simulink model "Unknown_Terrain_BOTS"  (R2018b)
settings: Solver=VariableStepAuto  StartTime=0.0  StopTime=10.0  RelTol=1e-3
model workspace: external: MATLAB File F:\Projects\Relative Localiztion\CAD models\Simulation\Unknown_Terrain_BOTS_DataFile.m (data not in the file)
values from neighbouring files (symbols this model uses):
  BOT1_pos = zeros(3,length(t))    [Tetrahedron_Based_Relative_Localization.m]
  bot1_transmitted = zeros(3,length(t))    [Transmission_Channal.m]
  BOT2_pos = zeros(3,length(t))    [Tetrahedron_Based_Relative_Localization.m]
  bot2_transmitted = zeros(3,length(t))    [Transmission_Channal.m]
  BOT3_pos = zeros(3,length(t))    [Tetrahedron_Based_Relative_Localization.m]
  bot3_transmitted = zeros(3,length(t))    [Transmission_Channal.m]
  BOT4_pos = zeros(3,length(t))    [Tetrahedron_Based_Relative_Localization.m]
  bot4_transmitted = zeros(3,length(t))    [Transmission_Channal.m]
undefined symbols (not defined in the file or in its folder): smiData, X, Y, Z
libraries: simulink x60, sm_lib x29, nesl_utility x25
(part 1 of 2)
settings Model: Creator=Yogesh  LastModifiedBy=Yogesh

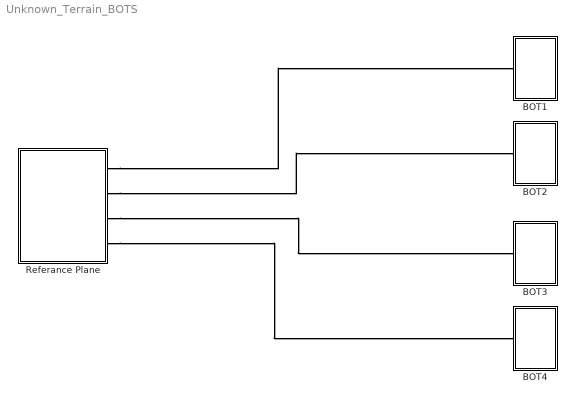
== system Unknown_Terrain_BOTS ==
  BOT1 : Subsystem
  BOT2 : Subsystem
  BOT3 : Subsystem
  BOT4 : Subsystem
  Referance Plane : Subsystem
  connections:
  Referance Plane/RConn1 -- BOT1/LConn1
  Referance Plane/RConn2 -- BOT2/LConn1
  Referance Plane/RConn3 -- BOT3/LConn1
  Referance Plane/RConn4 -- BOT4/LConn1

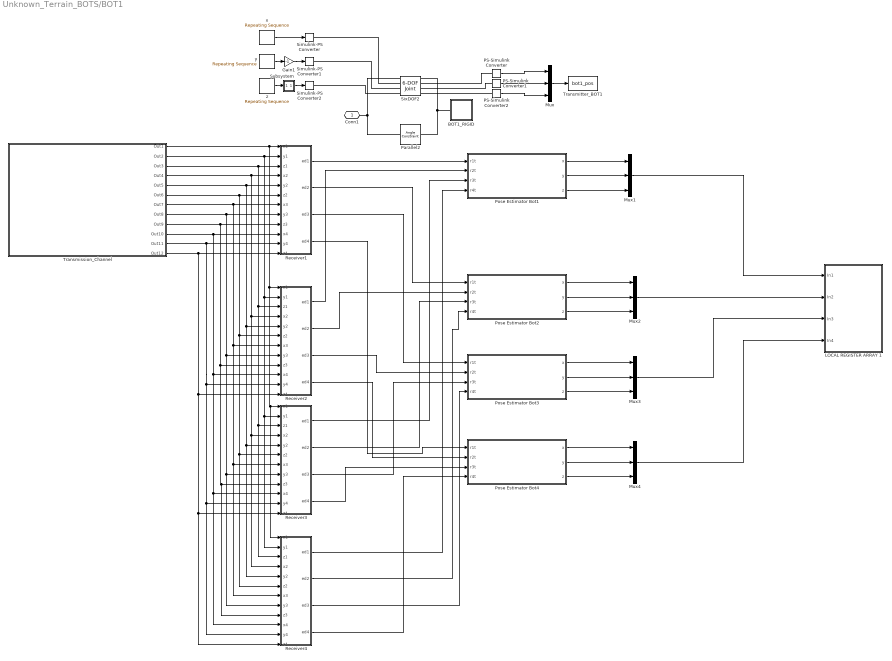
== system Unknown_Terrain_BOTS/BOT1 ==
  BOT1_RIGID : Subsystem
  Gain1 : Gain  Gain=-1
  LOCAL REGISTER ARRAY 1 : Subsystem
  Mux{,1..4} (5 alike) : Mux  Inputs=3
  PS-Simulink Converter : nesl_utility/PS-Simulink Converter  PhysicalDomain=network_engine_domain  SubClassName=ps_output  LeftPortType=input  RightPortType=output  PseudoPeriodic=off  Frequencies=[]  Unit=m  AffineConversion=off
  PS-Simulink Converter1 : nesl_utility/PS-Simulink Converter  PhysicalDomain=network_engine_domain  SubClassName=ps_output  LeftPortType=input  RightPortType=output  PseudoPeriodic=off  Frequencies=[]  Unit=m  AffineConversion=off
  PS-Simulink Converter2 : nesl_utility/PS-Simulink Converter  PhysicalDomain=network_engine_domain  SubClassName=ps_output  LeftPortType=input  RightPortType=output  PseudoPeriodic=off  Frequencies=[]  Unit=m  AffineConversion=off
  Parallel2 : sm_lib/Constraints/Angle Constraint  ConstraintType=Parallel  Angle=45  AngleUnits=deg  SenseSignedTorqueMagnitude=off  SenseTorque=off  SenseForce=off  WrenchDir=FollowerOnBase  WrenchFrame=BaseFrame
      settings: SourceProductName=Simscape Multibody  SourceProductBaseCode=MS
  Pose Estimator Bot1 : MATLAB Function  TreatAsAtomicUnit=on
  Pose Estimator Bot2 : MATLAB Function  TreatAsAtomicUnit=on
  Pose Estimator Bot3 : MATLAB Function  TreatAsAtomicUnit=on
  Pose Estimator Bot4 : MATLAB Function  TreatAsAtomicUnit=on
  Receiver1 : MATLAB Function  TreatAsAtomicUnit=on
  Receiver2 : MATLAB Function  TreatAsAtomicUnit=on
  Receiver3 : MATLAB Function  TreatAsAtomicUnit=on
  Receiver4 : MATLAB Function  TreatAsAtomicUnit=on
  Simulink-PS Converter : nesl_utility/Simulink-PS Converter  PhysicalDomain=network_engine_domain  SubClassName=ps_input  LeftPortType=input  RightPortType=output  PseudoPeriodic=off  Frequencies=[]  NoiseDistribution=none  NoiseParameters=[]  Unit=m  AffineConversion=off  FilteringAndDerivatives=filter  SimscapeFilterOrder=2  InputFilterTimeConstant=0.001  UdotUserProvided=0
  Simulink-PS Converter1 : nesl_utility/Simulink-PS Converter  PhysicalDomain=network_engine_domain  SubClassName=ps_input  LeftPortType=input  RightPortType=output  PseudoPeriodic=off  Frequencies=[]  NoiseDistribution=none  NoiseParameters=[]  Unit=m  AffineConversion=off  FilteringAndDerivatives=filter  SimscapeFilterOrder=2  InputFilterTimeConstant=0.001  UdotUserProvided=0
  Simulink-PS Converter2 : nesl_utility/Simulink-PS Converter  PhysicalDomain=network_engine_domain  SubClassName=ps_input  LeftPortType=input  RightPortType=output  PseudoPeriodic=off  Frequencies=[]  NoiseDistribution=none  NoiseParameters=[]  Unit=m  AffineConversion=off  FilteringAndDerivatives=filter  SimscapeFilterOrder=2  InputFilterTimeConstant=0.001  UdotUserProvided=0
  SixDOF2 : sm_lib/Joints/6-DOF Joint  SenseConstraintForce=off  SenseConstraintForceX=off  SenseConstraintForceY=off  SenseConstraintForceZ=off  SenseConstraintTorque=off  SenseConstraintTorqueX=off  SenseConstraintTorqueY=off  SenseConstraintTorqueZ=off  SenseTotalForce=off  SenseTotalForceX=off  SenseTotalForceY=off  SenseTotalForceZ=off  SenseTotalTorque=off  SenseTotalTorqueX=off  SenseTotalTorqueY=off  SenseTotalTorqueZ=off  CompositeWrenchDir=FollowerOnBase  CompositeWrenchFrame=BaseFrame  PxEquilibriumPosition=0  PxEquilibriumPositionUnits=m  PxSpringStiffness=0  PxSpringStiffnessUnits=N/m  PxDampingCoefficient=0  PxDampingCoefficientUnits=N/(m/s)  PxTorqueActuationMode=ComputedTorque  PxMotionActuationMode=InputMotion  PxSensePosition=on  PxSenseVelocity=off  PxSenseAcceleration=off  PxSenseTorqueForce=off  PxPositionTargetSpecify=on  PxPositionTargetPriority=Low  PxPositionTargetValue=smiData.SixDofJoint(3).Px.Pos  PxPositionTargetValueUnits=in  PxVelocityTargetSpecify=off  PxVelocityTargetPriority=High  PxVelocityTargetValue=0  PxVelocityTargetValueUnits=m/s  PyEquilibriumPosition=0  PyEquilibriumPositionUnits=m  PySpringStiffness=0  PySpringStiffnessUnits=N/m  PyDampingCoefficient=0  PyDampingCoefficientUnits=N/(m/s)  PyTorqueActuationMode=ComputedTorque  PyMotionActuationMode=InputMotion  PySensePosition=on  PySenseVelocity=off  PySenseAcceleration=off  PySenseTorqueForce=off  PyPositionTargetSpecify=on  PyPositionTargetPriority=Low  PyPositionTargetValue=smiData.SixDofJoint(3).Py.Pos  PyPositionTargetValueUnits=in  PyVelocityTargetSpecify=off  PyVelocityTargetPriority=High  PyVelocityTargetValue=0  PyVelocityTargetValueUnits=m/s  PzEquilibriumPosition=0  PzEquilibriumPositionUnits=m  PzSpringStiffness=0  PzSpringStiffnessUnits=N/m  PzDampingCoefficient=0  PzDampingCoefficientUnits=N/(m/s)  PzTorqueActuationMode=ComputedTorque  PzMotionActuationMode=InputMotion  PzSensePosition=on  PzSenseVelocity=off  PzSenseAcceleration=off  PzSenseTorqueForce=off  PzPositionTargetSpecify=on  PzPositionTargetPriority=Low  PzPositionTargetValue=smiData.SixDofJoint(3).Pz.Pos  PzPositionTargetValueUnits=in  PzVelocityTargetSpecify=off  PzVelocityTargetPriority=High  PzVelocityTargetValue=0  PzVelocityTargetValueUnits=m/s  SphDefPosRotationMethod=None  SphDefPosRotationAngleUnits=deg  SphDefPosRotationStandardAxis=+Z  SphDefPosRotationAngle=0.0  SphDefPosRotationArbitraryAxis=[0 0 1]  SphDefPosFollAlignAxisA=+X  SphDefPosBaseAlignAxisA=+Y  SphDefPosFollAlignAxisB=+Y  SphDefPosBaseAlignAxisB=+Z  SphDefPosRotationSequenceAxes=FollowerAxes  SphDefPosRotationSequence=XYX  SphDefPosRotationSequenceAngles=[0 0 0]  SphDefPosRotationSequenceAnglesUnits=deg  SphDefPosRotationMatrix=[1 0 0; 0 1 0; 0 0 1]  SphEqPosRotationMethod=None  SphEqPosRotationAngleUnits=deg  SphEqPosRotationStandardAxis=+Z  SphEqPosRotationAngle=0.0  SphEqPosRotationArbitraryAxis=[0 0 1]  SphEqPosFollAlignAxisA=+X  SphEqPosBaseAlignAxisA=+Y  SphEqPosFollAlignAxisB=+Y  SphEqPosBaseAlignAxisB=+Z  SphEqPosRotationSequenceAxes=FollowerAxes  SphEqPosRotationSequence=XYX  SphEqPosRotationSequenceAngles=[0 0 0]  SphEqPosRotationSequenceAnglesUnits=deg  SphEqPosRotationMatrix=[1 0 0; 0 1 0; 0 0 1]  SphSpringStiffness=0  SphSpringStiffnessUnits=N*m/rad  SphDampingCoefficient=0  SphDampingCoefficientUnits=N*m/(rad/s)  SphActuateTorqueX=off  SphActuateTorqueY=off  SphActuateTorqueZ=off  SphActuateTorque=off  SphTorqueActuationMode=NoTorque  SphMotionActuationMode=ComputedMotion  SphActuationFrame=BaseFrame  SphSensePosition=off  SphSenseVelocityX=off  SphSenseVelocityY=off  SphSenseVelocityZ=off  SphSenseVelocity=off  SphSenseAccelerationX=off  SphSenseAccelerationY=off  SphSenseAccelerationZ=off  SphSenseAcceleration=off  SphSenseTorqueX=off  SphSenseTorqueY=off  SphSenseTorqueZ=off  SphSenseTorqueForce=off  SphSensingFrame=FollowerFrame  SphPositionTargetRotationMethod=ArbitraryAxis  SphPositionTargetRotationAngleUnits=deg  SphPositionTargetRotationStandardAxis=+Z  SphPositionTargetRotationAngle=smiData.SixDofJoint(3).S.Pos.Angle  SphPositionTargetRotationArbitraryAxis=smiData.SixDofJoint(3).S.Pos.Axis  SphPositionTargetFollAlignAxisA=+X  SphPositionTargetBaseAlignAxisA=+Y  SphPositionTargetFollAlignAxisB=+Y  SphPositionTargetBaseAlignAxisB=+Z  SphPositionTargetRotationSequenceAxes=FollowerAxes  SphPositionTargetRotationSequence=XYX  SphPositionTargetRotationSequenceAngles=[0 0 0]  SphPositionTargetRotationSequenceAnglesUnits=deg  SphPositionTargetRotationMatrix=[1 0 0; 0 1 0; 0 0 1]  SphPositionTargetSpecify=on  SphPositionTargetPriority=Low  SphVelocityTargetValue=[0 0 0]  SphVelocityTargetValueUnits=deg/s  SphVelocityTargetSpecify=off  SphVelocityTargetPriority=High  SphVelocityTargetInFollowerFrame=on
  Subsystem : Subsystem
  Transmission_Channel : Subsystem
  Transmitter_BOT1 : ToWorkspace  VariableName=bot1_pos  SampleTime=-1
  x : simulink/Sources/Repeating Sequence  rep_seq_t=t  rep_seq_y=BOT1_pos(1,:)
  y : simulink/Sources/Repeating Sequence  rep_seq_t=t  rep_seq_y=BOT1_pos(2,:)
  z : simulink/Sources/Repeating Sequence  rep_seq_t=t  rep_seq_y=BOT1_pos(3,:)
  Conn1 : PMIOPort  Side=Left
  wires:
  y/1 -> Gain1/1
  z/1 -> Subsystem/1(1)
  Subsystem/1(2) -> Simulink-PS Converter2/1
  x/1 -> Simulink-PS Converter/1
  Gain1/1 -> Simulink-PS Converter1/1
  Mux/1 -> Transmitter_BOT1/1
  PS-Simulink Converter/1 -> Mux/1
  PS-Simulink Converter1/1 -> Mux/2
  PS-Simulink Converter2/1 -> Mux/3
  Receiver4/4(ed4) -> Pose Estimator Bot4/4(r4t)
  Pose Estimator Bot4/1(x) -> Mux4/1
  Pose Estimator Bot3/3(z) -> Mux3/3
  Pose Estimator Bot1/2(y) -> Mux1/2
  Pose Estimator Bot2/2(y) -> Mux2/2
  Pose Estimator Bot1/3(z) -> Mux1/3
  Receiver3/4(ed4) -> Pose Estimator Bot4/3(r3t)
  Pose Estimator Bot4/2(y) -> Mux4/2
  Pose Estimator Bot1/1(x) -> Mux1/1
  Receiver2/4(ed4) -> Pose Estimator Bot4/2(r2t)
  Receiver3/2(ed2) -> Pose Estimator Bot2/3(r3t)
  Pose Estimator Bot2/3(z) -> Mux2/3
  Pose Estimator Bot2/1(x) -> Mux2/1
  Pose Estimator Bot3/2(y) -> Mux3/2
  Receiver4/3(ed3) -> Pose Estimator Bot3/4(r4t)
  Receiver4/2(ed2) -> Pose Estimator Bot2/4(r4t)
  Pose Estimator Bot4/3(z) -> Mux4/3
  Transmission_Channel/12(Out12) -> Receiver4/12(z4), Receiver3/12(z4), Receiver2/12(z4), Receiver1/12(z4)
  Transmission_Channel/11(Out11) -> Receiver4/11(y4), Receiver3/11(y4), Receiver2/11(y4), Receiver1/11(y4)
  Transmission_Channel/7(Out7) -> Receiver2/7(x3), Receiver4/7(x3), Receiver3/7(x3), Receiver1/7(x3)
  Pose Estimator Bot3/1(x) -> Mux3/1
  Transmission_Channel/10(Out10) -> Receiver4/10(x4), Receiver3/10(x4), Receiver2/10(x4), Receiver1/10(x4)
  Transmission_Channel/6(Out6) -> Receiver2/6(z2), Receiver4/6(z2), Receiver3/6(z2), Receiver1/6(z2)
  Transmission_Channel/9(Out9) -> Receiver4/9(z3), Receiver3/9(z3), Receiver2/9(z3), Receiver1/9(z3)
  Transmission_Channel/8(Out8) -> Receiver4/8(y3), Receiver3/8(y3), Receiver2/8(y3), Receiver1/8(y3)
  Transmission_Channel/4(Out4) -> Receiver4/4(x2), Receiver3/4(x2), Receiver2/4(x2), Receiver1/4(x2)
  Transmission_Channel/1(Out1) -> Receiver4/1(x1), Receiver3/1(x1), Receiver2/1(x1), Receiver1/1(x1)
  Transmission_Channel/5(Out5) -> Receiver4/5(y2), Receiver3/5(y2), Receiver2/5(y2), Receiver1/5(y2)
  Transmission_Channel/2(Out2) -> Receiver4/2(y1), Receiver3/2(y1), Receiver2/2(y1), Receiver1/2(y1)
  Receiver1/1(ed1) -> Pose Estimator Bot1/1(r1t)
  Mux3/1 -> LOCAL REGISTER ARRAY 1/3(In3)
  Mux4/1 -> LOCAL REGISTER ARRAY 1/4(In4)
  Mux1/1 -> LOCAL REGISTER ARRAY 1/1(In1)
  Receiver1/2(ed2) -> Pose Estimator Bot2/1(r1t)
  Receiver2/1(ed1) -> Pose Estimator Bot1/2(r2t)
  Mux2/1 -> LOCAL REGISTER ARRAY 1/2(In2)
  Receiver3/1(ed1) -> Pose Estimator Bot1/3(r3t)
  Receiver1/4(ed4) -> Pose Estimator Bot4/1(r1t)
  Receiver1/3(ed3) -> Pose Estimator Bot3/1(r1t)
  Receiver3/3(ed3) -> Pose Estimator Bot3/3(r3t)
  Transmission_Channel/3(Out3) -> Receiver4/3(z1), Receiver3/3(z1), Receiver2/3(z1), Receiver1/3(z1)
  Receiver2/3(ed3) -> Pose Estimator Bot3/2(r2t)
  Receiver2/2(ed2) -> Pose Estimator Bot2/2(r2t)
  Receiver4/1(ed1) -> Pose Estimator Bot1/4(r4t)
  connections:
  Conn1/RConn1 -- SixDOF2/LConn1 -- Parallel2/LConn1
  Parallel2/RConn1 -- BOT1_RIGID/LConn1 -- SixDOF2/RConn1
  SixDOF2/LConn3 -- Simulink-PS Converter1/RConn1
  SixDOF2/LConn2 -- Simulink-PS Converter/RConn1
  SixDOF2/LConn4 -- Simulink-PS Converter2/RConn1
  PS-Simulink Converter/LConn1 -- SixDOF2/RConn2
  PS-Simulink Converter1/LConn1 -- SixDOF2/RConn3
  PS-Simulink Converter2/LConn1 -- SixDOF2/RConn4

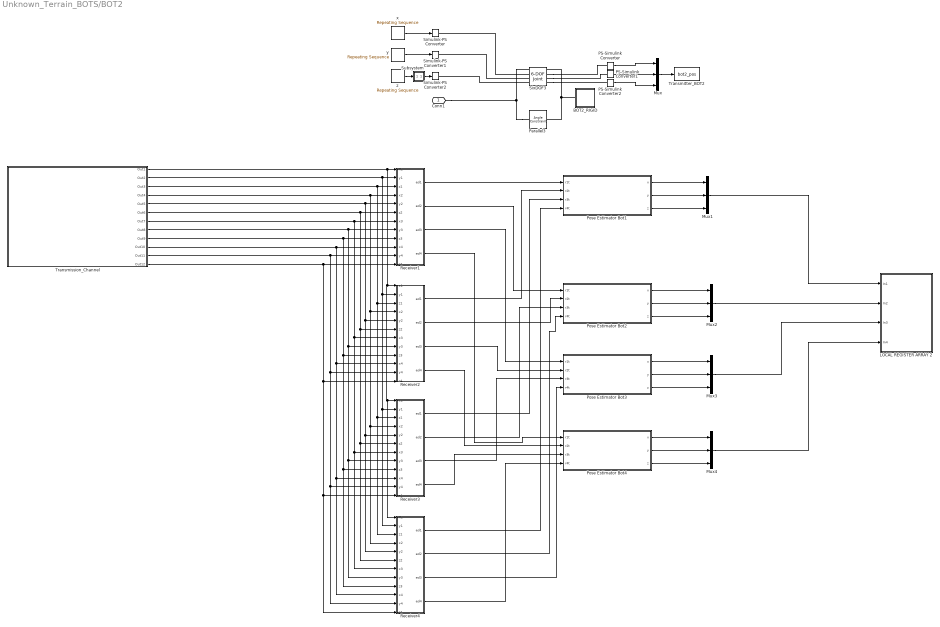
== system Unknown_Terrain_BOTS/BOT2 ==
  BOT2_RIGID : Subsystem
  LOCAL REGISTER ARRAY 2 : Subsystem
  Mux{,1..4} (5 alike) : Mux  Inputs=3
  PS-Simulink Converter : nesl_utility/PS-Simulink Converter  PhysicalDomain=network_engine_domain  SubClassName=ps_output  LeftPortType=input  RightPortType=output  PseudoPeriodic=off  Frequencies=[]  Unit=m  AffineConversion=off
  PS-Simulink Converter1 : nesl_utility/PS-Simulink Converter  PhysicalDomain=network_engine_domain  SubClassName=ps_output  LeftPortType=input  RightPortType=output  PseudoPeriodic=off  Frequencies=[]  Unit=m  AffineConversion=off
  PS-Simulink Converter2 : nesl_utility/PS-Simulink Converter  PhysicalDomain=network_engine_domain  SubClassName=ps_output  LeftPortType=input  RightPortType=output  PseudoPeriodic=off  Frequencies=[]  Unit=m  AffineConversion=off
  Parallel3 : sm_lib/Constraints/Angle Constraint  ConstraintType=Parallel  Angle=45  AngleUnits=deg  SenseSignedTorqueMagnitude=off  SenseTorque=off  SenseForce=off  WrenchDir=FollowerOnBase  WrenchFrame=BaseFrame
      settings: SourceProductName=Simscape Multibody  SourceProductBaseCode=MS
  Pose Estimator Bot1 : MATLAB Function  TreatAsAtomicUnit=on
  Pose Estimator Bot2 : MATLAB Function  TreatAsAtomicUnit=on
  Pose Estimator Bot3 : MATLAB Function  TreatAsAtomicUnit=on
  Pose Estimator Bot4 : MATLAB Function  TreatAsAtomicUnit=on
  Receiver1 : MATLAB Function  TreatAsAtomicUnit=on
  Receiver2 : MATLAB Function  TreatAsAtomicUnit=on
  Receiver3 : MATLAB Function  TreatAsAtomicUnit=on
  Receiver4 : MATLAB Function  TreatAsAtomicUnit=on
  Simulink-PS Converter : nesl_utility/Simulink-PS Converter  PhysicalDomain=network_engine_domain  SubClassName=ps_input  LeftPortType=input  RightPortType=output  PseudoPeriodic=off  Frequencies=[]  NoiseDistribution=none  NoiseParameters=[]  Unit=m  AffineConversion=off  FilteringAndDerivatives=filter  SimscapeFilterOrder=2  InputFilterTimeConstant=0.001  UdotUserProvided=0
  Simulink-PS Converter1 : nesl_utility/Simulink-PS Converter  PhysicalDomain=network_engine_domain  SubClassName=ps_input  LeftPortType=input  RightPortType=output  PseudoPeriodic=off  Frequencies=[]  NoiseDistribution=none  NoiseParameters=[]  Unit=m  AffineConversion=off  FilteringAndDerivatives=filter  SimscapeFilterOrder=2  InputFilterTimeConstant=0.001  UdotUserProvided=0
  Simulink-PS Converter2 : nesl_utility/Simulink-PS Converter  PhysicalDomain=network_engine_domain  SubClassName=ps_input  LeftPortType=input  RightPortType=output  PseudoPeriodic=off  Frequencies=[]  NoiseDistribution=none  NoiseParameters=[]  Unit=m  AffineConversion=off  FilteringAndDerivatives=filter  SimscapeFilterOrder=2  InputFilterTimeConstant=0.001  UdotUserProvided=0
  SixDOF3 : sm_lib/Joints/6-DOF Joint  SenseConstraintForce=off  SenseConstraintForceX=off  SenseConstraintForceY=off  SenseConstraintForceZ=off  SenseConstraintTorque=off  SenseConstraintTorqueX=off  SenseConstraintTorqueY=off  SenseConstraintTorqueZ=off  SenseTotalForce=off  SenseTotalForceX=off  SenseTotalForceY=off  SenseTotalForceZ=off  SenseTotalTorque=off  SenseTotalTorqueX=off  SenseTotalTorqueY=off  SenseTotalTorqueZ=off  CompositeWrenchDir=FollowerOnBase  CompositeWrenchFrame=BaseFrame  PxEquilibriumPosition=0  PxEquilibriumPositionUnits=m  PxSpringStiffness=0  PxSpringStiffnessUnits=N/m  PxDampingCoefficient=0  PxDampingCoefficientUnits=N/(m/s)  PxTorqueActuationMode=ComputedTorque  PxMotionActuationMode=InputMotion  PxSensePosition=on  PxSenseVelocity=off  PxSenseAcceleration=off  PxSenseTorqueForce=off  PxPositionTargetSpecify=on  PxPositionTargetPriority=Low  PxPositionTargetValue=smiData.SixDofJoint(4).Px.Pos  PxPositionTargetValueUnits=in  PxVelocityTargetSpecify=off  PxVelocityTargetPriority=High  PxVelocityTargetValue=0  PxVelocityTargetValueUnits=m/s  PyEquilibriumPosition=0  PyEquilibriumPositionUnits=m  PySpringStiffness=0  PySpringStiffnessUnits=N/m  PyDampingCoefficient=0  PyDampingCoefficientUnits=N/(m/s)  PyTorqueActuationMode=ComputedTorque  PyMotionActuationMode=InputMotion  PySensePosition=on  PySenseVelocity=off  PySenseAcceleration=off  PySenseTorqueForce=off  PyPositionTargetSpecify=on  PyPositionTargetPriority=Low  PyPositionTargetValue=smiData.SixDofJoint(4).Py.Pos  PyPositionTargetValueUnits=in  PyVelocityTargetSpecify=off  PyVelocityTargetPriority=High  PyVelocityTargetValue=0  PyVelocityTargetValueUnits=m/s  PzEquilibriumPosition=0  PzEquilibriumPositionUnits=m  PzSpringStiffness=0  PzSpringStiffnessUnits=N/m  PzDampingCoefficient=0  PzDampingCoefficientUnits=N/(m/s)  PzTorqueActuationMode=ComputedTorque  PzMotionActuationMode=InputMotion  PzSensePosition=on  PzSenseVelocity=off  PzSenseAcceleration=off  PzSenseTorqueForce=off  PzPositionTargetSpecify=on  PzPositionTargetPriority=Low  PzPositionTargetValue=smiData.SixDofJoint(4).Pz.Pos  PzPositionTargetValueUnits=in  PzVelocityTargetSpecify=off  PzVelocityTargetPriority=High  PzVelocityTargetValue=0  PzVelocityTargetValueUnits=m/s  SphDefPosRotationMethod=None  SphDefPosRotationAngleUnits=deg  SphDefPosRotationStandardAxis=+Z  SphDefPosRotationAngle=0.0  SphDefPosRotationArbitraryAxis=[0 0 1]  SphDefPosFollAlignAxisA=+X  SphDefPosBaseAlignAxisA=+Y  SphDefPosFollAlignAxisB=+Y  SphDefPosBaseAlignAxisB=+Z  SphDefPosRotationSequenceAxes=FollowerAxes  SphDefPosRotationSequence=XYX  SphDefPosRotationSequenceAngles=[0 0 0]  SphDefPosRotationSequenceAnglesUnits=deg  SphDefPosRotationMatrix=[1 0 0; 0 1 0; 0 0 1]  SphEqPosRotationMethod=None  SphEqPosRotationAngleUnits=deg  SphEqPosRotationStandardAxis=+Z  SphEqPosRotationAngle=0.0  SphEqPosRotationArbitraryAxis=[0 0 1]  SphEqPosFollAlignAxisA=+X  SphEqPosBaseAlignAxisA=+Y  SphEqPosFollAlignAxisB=+Y  SphEqPosBaseAlignAxisB=+Z  SphEqPosRotationSequenceAxes=FollowerAxes  SphEqPosRotationSequence=XYX  SphEqPosRotationSequenceAngles=[0 0 0]  SphEqPosRotationSequenceAnglesUnits=deg  SphEqPosRotationMatrix=[1 0 0; 0 1 0; 0 0 1]  SphSpringStiffness=0  SphSpringStiffnessUnits=N*m/rad  SphDampingCoefficient=0  SphDampingCoefficientUnits=N*m/(rad/s)  SphActuateTorqueX=off  SphActuateTorqueY=off  SphActuateTorqueZ=off  SphActuateTorque=off  SphTorqueActuationMode=NoTorque  SphMotionActuationMode=ComputedMotion  SphActuationFrame=BaseFrame  SphSensePosition=off  SphSenseVelocityX=off  SphSenseVelocityY=off  SphSenseVelocityZ=off  SphSenseVelocity=off  SphSenseAccelerationX=off  SphSenseAccelerationY=off  SphSenseAccelerationZ=off  SphSenseAcceleration=off  SphSenseTorqueX=off  SphSenseTorqueY=off  SphSenseTorqueZ=off  SphSenseTorqueForce=off  SphSensingFrame=FollowerFrame  SphPositionTargetRotationMethod=ArbitraryAxis  SphPositionTargetRotationAngleUnits=deg  SphPositionTargetRotationStandardAxis=+Z  SphPositionTargetRotationAngle=smiData.SixDofJoint(4).S.Pos.Angle  SphPositionTargetRotationArbitraryAxis=smiData.SixDofJoint(4).S.Pos.Axis  SphPositionTargetFollAlignAxisA=+X  SphPositionTargetBaseAlignAxisA=+Y  SphPositionTargetFollAlignAxisB=+Y  SphPositionTargetBaseAlignAxisB=+Z  SphPositionTargetRotationSequenceAxes=FollowerAxes  SphPositionTargetRotationSequence=XYX  SphPositionTargetRotationSequenceAngles=[0 0 0]  SphPositionTargetRotationSequenceAnglesUnits=deg  SphPositionTargetRotationMatrix=[1 0 0; 0 1 0; 0 0 1]  SphPositionTargetSpecify=on  SphPositionTargetPriority=Low  SphVelocityTargetValue=[0 0 0]  SphVelocityTargetValueUnits=deg/s  SphVelocityTargetSpecify=off  SphVelocityTargetPriority=High  SphVelocityTargetInFollowerFrame=on
  Subsystem : Subsystem
  Transmission_Channel : Subsystem
  Transmitter_BOT2 : ToWorkspace  VariableName=bot2_pos  SampleTime=-1
  x : simulink/Sources/Repeating Sequence  rep_seq_t=t  rep_seq_y=BOT2_pos(1,:)
  y : simulink/Sources/Repeating Sequence  rep_seq_t=t  rep_seq_y=BOT2_pos(2,:)
  z : simulink/Sources/Repeating Sequence  rep_seq_t=t  rep_seq_y=BOT2_pos(3,:)
  Conn1 : PMIOPort  Side=Left
  wires:
  x/1 -> Simulink-PS Converter/1
  y/1 -> Simulink-PS Converter1/1
  z/1 -> Subsystem/1(1)
  Subsystem/1(2) -> Simulink-PS Converter2/1
  PS-Simulink Converter1/1 -> Mux/2
  PS-Simulink Converter2/1 -> Mux/3
  PS-Simulink Converter/1 -> Mux/1
  Mux/1 -> Transmitter_BOT2/1
  Pose Estimator Bot4/2(y) -> Mux4/2
  Pose Estimator Bot1/3(z) -> Mux1/3
  Pose Estimator Bot2/2(y) -> Mux2/2
  Pose Estimator Bot1/2(y) -> Mux1/2
  Pose Estimator Bot3/3(z) -> Mux3/3
  Receiver4/4(ed4) -> Pose Estimator Bot4/4(r4t)
  Transmission_Channel/11(Out11) -> Receiver4/11(y4), Receiver3/11(y4), Receiver2/11(y4), Receiver1/11(y4)
  Transmission_Channel/12(Out12) -> Receiver4/12(z4), Receiver3/12(z4), Receiver2/12(z4), Receiver1/12(z4)
  Pose Estimator Bot4/3(z) -> Mux4/3
  Receiver4/2(ed2) -> Pose Estimator Bot2/4(r4t)
  Pose Estimator Bot3/2(y) -> Mux3/2
  Pose Estimator Bot2/1(x) -> Mux2/1
  Pose Estimator Bot2/3(z) -> Mux2/3
  Pose Estimator Bot4/1(x) -> Mux4/1
  Receiver2/4(ed4) -> Pose Estimator Bot4/2(r2t)
  Pose Estimator Bot1/1(x) -> Mux1/1
  Receiver2/2(ed2) -> Pose Estimator Bot2/2(r2t)
  Receiver2/3(ed3) -> Pose Estimator Bot3/2(r2t)
  Receiver3/4(ed4) -> Pose Estimator Bot4/3(r3t)
  Transmission_Channel/3(Out3) -> Receiver4/3(z1), Receiver3/3(z1), Receiver2/3(z1), Receiver1/3(z1)
  Receiver3/3(ed3) -> Pose Estimator Bot3/3(r3t)
  Receiver3/1(ed1) -> Pose Estimator Bot1/3(r3t)
  Pose Estimator Bot3/1(x) -> Mux3/1
  Transmission_Channel/7(Out7) -> Receiver2/7(x3), Receiver4/7(x3), Receiver3/7(x3), Receiver1/7(x3)
  Receiver2/1(ed1) -> Pose Estimator Bot1/2(r2t)
  Receiver1/2(ed2) -> Pose Estimator Bot2/1(r1t)
  Mux4/1 -> LOCAL REGISTER ARRAY 2/4(In4)
  Transmission_Channel/9(Out9) -> Receiver4/9(z3), Receiver3/9(z3), Receiver2/9(z3), Receiver1/9(z3)
  Mux1/1 -> LOCAL REGISTER ARRAY 2/1(In1)
  Transmission_Channel/2(Out2) -> Receiver4/2(y1), Receiver3/2(y1), Receiver2/2(y1), Receiver1/2(y1)
  Transmission_Channel/6(Out6) -> Receiver2/6(z2), Receiver4/6(z2), Receiver3/6(z2), Receiver1/6(z2)
  Receiver1/3(ed3) -> Pose Estimator Bot3/1(r1t)
  Mux2/1 -> LOCAL REGISTER ARRAY 2/2(In2)
  Transmission_Channel/5(Out5) -> Receiver4/5(y2), Receiver3/5(y2), Receiver2/5(y2), Receiver1/5(y2)
  Receiver4/1(ed1) -> Pose Estimator Bot1/4(r4t)
  Transmission_Channel/10(Out10) -> Receiver4/10(x4), Receiver3/10(x4), Receiver2/10(x4), Receiver1/10(x4)
  Transmission_Channel/4(Out4) -> Receiver4/4(x2), Receiver3/4(x2), Receiver2/4(x2), Receiver1/4(x2)
  Receiver1/4(ed4) -> Pose Estimator Bot4/1(r1t)
  Receiver1/1(ed1) -> Pose Estimator Bot1/1(r1t)
  Receiver4/3(ed3) -> Pose Estimator Bot3/4(r4t)
  Mux3/1 -> LOCAL REGISTER ARRAY 2/3(In3)
  Transmission_Channel/8(Out8) -> Receiver4/8(y3), Receiver3/8(y3), Receiver2/8(y3), Receiver1/8(y3)
  Transmission_Channel/1(Out1) -> Receiver4/1(x1), Receiver3/1(x1), Receiver2/1(x1), Receiver1/1(x1)
  Receiver3/2(ed2) -> Pose Estimator Bot2/3(r3t)
  connections:
  Parallel3/LConn1 -- SixDOF3/LConn1 -- Conn1/RConn1
  Parallel3/RConn1 -- SixDOF3/RConn1 -- BOT2_RIGID/LConn1
  SixDOF3/LConn4 -- Simulink-PS Converter2/RConn1
  SixDOF3/LConn2 -- Simulink-PS Converter/RConn1
  SixDOF3/LConn3 -- Simulink-PS Converter1/RConn1
  SixDOF3/RConn4 -- PS-Simulink Converter2/LConn1
  SixDOF3/RConn3 -- PS-Simulink Converter1/LConn1
  SixDOF3/RConn2 -- PS-Simulink Converter/LConn1

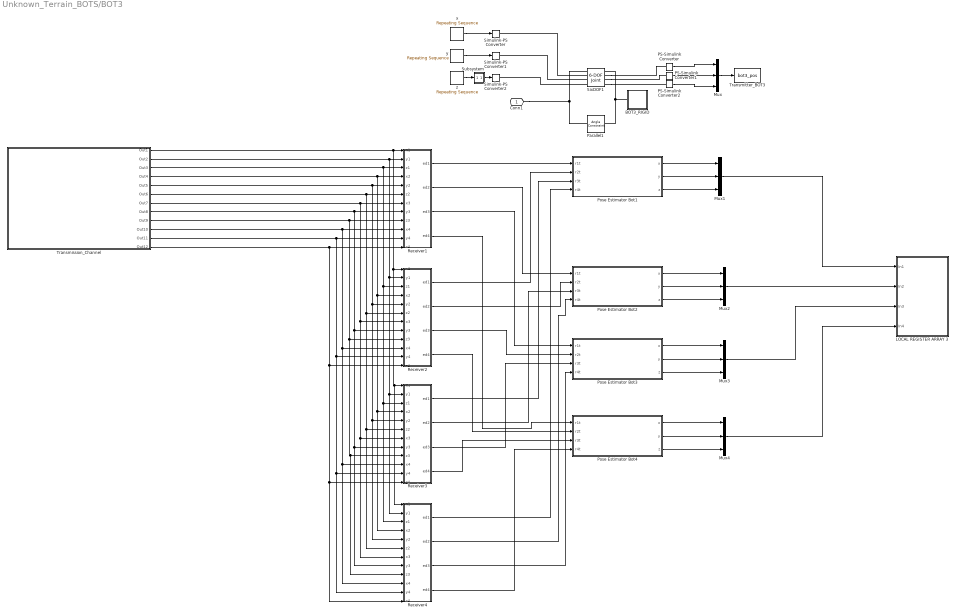
== system Unknown_Terrain_BOTS/BOT3 ==
  BOT3_RIGID : Subsystem
  LOCAL REGISTER ARRAY 3 : Subsystem
  Mux{,1..4} (5 alike) : Mux  Inputs=3
  PS-Simulink Converter : nesl_utility/PS-Simulink Converter  PhysicalDomain=network_engine_domain  SubClassName=ps_output  LeftPortType=input  RightPortType=output  PseudoPeriodic=off  Frequencies=[]  Unit=m  AffineConversion=off
  PS-Simulink Converter1 : nesl_utility/PS-Simulink Converter  PhysicalDomain=network_engine_domain  SubClassName=ps_output  LeftPortType=input  RightPortType=output  PseudoPeriodic=off  Frequencies=[]  Unit=m  AffineConversion=off
  PS-Simulink Converter2 : nesl_utility/PS-Simulink Converter  PhysicalDomain=network_engine_domain  SubClassName=ps_output  LeftPortType=input  RightPortType=output  PseudoPeriodic=off  Frequencies=[]  Unit=m  AffineConversion=off
  Parallel1 : sm_lib/Constraints/Angle Constraint  ConstraintType=Parallel  Angle=45  AngleUnits=deg  SenseSignedTorqueMagnitude=off  SenseTorque=off  SenseForce=off  WrenchDir=FollowerOnBase  WrenchFrame=BaseFrame
      settings: SourceProductName=Simscape Multibody  SourceProductBaseCode=MS
  Pose Estimator Bot1 : MATLAB Function  TreatAsAtomicUnit=on
  Pose Estimator Bot2 : MATLAB Function  TreatAsAtomicUnit=on
  Pose Estimator Bot3 : MATLAB Function  TreatAsAtomicUnit=on
  Pose Estimator Bot4 : MATLAB Function  TreatAsAtomicUnit=on
  Receiver1 : MATLAB Function  TreatAsAtomicUnit=on
  Receiver2 : MATLAB Function  TreatAsAtomicUnit=on
  Receiver3 : MATLAB Function  TreatAsAtomicUnit=on
  Receiver4 : MATLAB Function  TreatAsAtomicUnit=on
  Simulink-PS Converter : nesl_utility/Simulink-PS Converter  PhysicalDomain=network_engine_domain  SubClassName=ps_input  LeftPortType=input  RightPortType=output  PseudoPeriodic=off  Frequencies=[]  NoiseDistribution=none  NoiseParameters=[]  Unit=m  AffineConversion=off  FilteringAndDerivatives=filter  SimscapeFilterOrder=2  InputFilterTimeConstant=0.001  UdotUserProvided=0
  Simulink-PS Converter1 : nesl_utility/Simulink-PS Converter  PhysicalDomain=network_engine_domain  SubClassName=ps_input  LeftPortType=input  RightPortType=output  PseudoPeriodic=off  Frequencies=[]  NoiseDistribution=none  NoiseParameters=[]  Unit=m  AffineConversion=off  FilteringAndDerivatives=filter  SimscapeFilterOrder=2  InputFilterTimeConstant=0.001  UdotUserProvided=0
  Simulink-PS Converter2 : nesl_utility/Simulink-PS Converter  PhysicalDomain=network_engine_domain  SubClassName=ps_input  LeftPortType=input  RightPortType=output  PseudoPeriodic=off  Frequencies=[]  NoiseDistribution=none  NoiseParameters=[]  Unit=m  AffineConversion=off  FilteringAndDerivatives=filter  SimscapeFilterOrder=2  InputFilterTimeConstant=0.001  UdotUserProvided=0
  SixDOF1 : sm_lib/Joints/6-DOF Joint  SenseConstraintForce=off  SenseConstraintForceX=off  SenseConstraintForceY=off  SenseConstraintForceZ=off  SenseConstraintTorque=off  SenseConstraintTorqueX=off  SenseConstraintTorqueY=off  SenseConstraintTorqueZ=off  SenseTotalForce=off  SenseTotalForceX=off  SenseTotalForceY=off  SenseTotalForceZ=off  SenseTotalTorque=off  SenseTotalTorqueX=off  SenseTotalTorqueY=off  SenseTotalTorqueZ=off  CompositeWrenchDir=FollowerOnBase  CompositeWrenchFrame=BaseFrame  PxEquilibriumPosition=0  PxEquilibriumPositionUnits=m  PxSpringStiffness=0  PxSpringStiffnessUnits=N/m  PxDampingCoefficient=0  PxDampingCoefficientUnits=N/(m/s)  PxTorqueActuationMode=ComputedTorque  PxMotionActuationMode=InputMotion  PxSensePosition=on  PxSenseVelocity=off  PxSenseAcceleration=off  PxSenseTorqueForce=off  PxPositionTargetSpecify=on  PxPositionTargetPriority=Low  PxPositionTargetValue=smiData.SixDofJoint(2).Px.Pos  PxPositionTargetValueUnits=in  PxVelocityTargetSpecify=off  PxVelocityTargetPriority=High  PxVelocityTargetValue=0  PxVelocityTargetValueUnits=m/s  PyEquilibriumPosition=0  PyEquilibriumPositionUnits=m  PySpringStiffness=0  PySpringStiffnessUnits=N/m  PyDampingCoefficient=0  PyDampingCoefficientUnits=N/(m/s)  PyTorqueActuationMode=ComputedTorque  PyMotionActuationMode=InputMotion  PySensePosition=on  PySenseVelocity=off  PySenseAcceleration=off  PySenseTorqueForce=off  PyPositionTargetSpecify=on  PyPositionTargetPriority=Low  PyPositionTargetValue=smiData.SixDofJoint(2).Py.Pos  PyPositionTargetValueUnits=in  PyVelocityTargetSpecify=off  PyVelocityTargetPriority=High  PyVelocityTargetValue=0  PyVelocityTargetValueUnits=m/s  PzEquilibriumPosition=0  PzEquilibriumPositionUnits=m  PzSpringStiffness=0  PzSpringStiffnessUnits=N/m  PzDampingCoefficient=0  PzDampingCoefficientUnits=N/(m/s)  PzTorqueActuationMode=ComputedTorque  PzMotionActuationMode=InputMotion  PzSensePosition=on  PzSenseVelocity=off  PzSenseAcceleration=off  PzSenseTorqueForce=off  PzPositionTargetSpecify=on  PzPositionTargetPriority=Low  PzPositionTargetValue=smiData.SixDofJoint(2).Pz.Pos  PzPositionTargetValueUnits=in  PzVelocityTargetSpecify=off  PzVelocityTargetPriority=High  PzVelocityTargetValue=0  PzVelocityTargetValueUnits=m/s  SphDefPosRotationMethod=None  SphDefPosRotationAngleUnits=deg  SphDefPosRotationStandardAxis=+Z  SphDefPosRotationAngle=0.0  SphDefPosRotationArbitraryAxis=[0 0 1]  SphDefPosFollAlignAxisA=+X  SphDefPosBaseAlignAxisA=+Y  SphDefPosFollAlignAxisB=+Y  SphDefPosBaseAlignAxisB=+Z  SphDefPosRotationSequenceAxes=FollowerAxes  SphDefPosRotationSequence=XYX  SphDefPosRotationSequenceAngles=[0 0 0]  SphDefPosRotationSequenceAnglesUnits=deg  SphDefPosRotationMatrix=[1 0 0; 0 1 0; 0 0 1]  SphEqPosRotationMethod=None  SphEqPosRotationAngleUnits=deg  SphEqPosRotationStandardAxis=+Z  SphEqPosRotationAngle=0.0  SphEqPosRotationArbitraryAxis=[0 0 1]  SphEqPosFollAlignAxisA=+X  SphEqPosBaseAlignAxisA=+Y  SphEqPosFollAlignAxisB=+Y  SphEqPosBaseAlignAxisB=+Z  SphEqPosRotationSequenceAxes=FollowerAxes  SphEqPosRotationSequence=XYX  SphEqPosRotationSequenceAngles=[0 0 0]  SphEqPosRotationSequenceAnglesUnits=deg  SphEqPosRotationMatrix=[1 0 0; 0 1 0; 0 0 1]  SphSpringStiffness=0  SphSpringStiffnessUnits=N*m/rad  SphDampingCoefficient=0  SphDampingCoefficientUnits=N*m/(rad/s)  SphActuateTorqueX=off  SphActuateTorqueY=off  SphActuateTorqueZ=off  SphActuateTorque=off  SphTorqueActuationMode=NoTorque  SphMotionActuationMode=ComputedMotion  SphActuationFrame=BaseFrame  SphSensePosition=off  SphSenseVelocityX=off  SphSenseVelocityY=off  SphSenseVelocityZ=off  SphSenseVelocity=off  SphSenseAccelerationX=off  SphSenseAccelerationY=off  SphSenseAccelerationZ=off  SphSenseAcceleration=off  SphSenseTorqueX=off  SphSenseTorqueY=off  SphSenseTorqueZ=off  SphSenseTorqueForce=off  SphSensingFrame=FollowerFrame  SphPositionTargetRotationMethod=ArbitraryAxis  SphPositionTargetRotationAngleUnits=deg  SphPositionTargetRotationStandardAxis=+Z  SphPositionTargetRotationAngle=smiData.SixDofJoint(2).S.Pos.Angle  SphPositionTargetRotationArbitraryAxis=smiData.SixDofJoint(2).S.Pos.Axis  SphPositionTargetFollAlignAxisA=+X  SphPositionTargetBaseAlignAxisA=+Y  SphPositionTargetFollAlignAxisB=+Y  SphPositionTargetBaseAlignAxisB=+Z  SphPositionTargetRotationSequenceAxes=FollowerAxes  SphPositionTargetRotationSequence=XYX  SphPositionTargetRotationSequenceAngles=[0 0 0]  SphPositionTargetRotationSequenceAnglesUnits=deg  SphPositionTargetRotationMatrix=[1 0 0; 0 1 0; 0 0 1]  SphPositionTargetSpecify=on  SphPositionTargetPriority=Low  SphVelocityTargetValue=[0 0 0]  SphVelocityTargetValueUnits=deg/s  SphVelocityTargetSpecify=off  SphVelocityTargetPriority=High  SphVelocityTargetInFollowerFrame=on
  Subsystem : Subsystem
  Transmission_Channel : Subsystem
  Transmitter_BOT3 : ToWorkspace  VariableName=bot3_pos  SampleTime=-1
  x : simulink/Sources/Repeating Sequence  rep_seq_t=t  rep_seq_y=BOT3_pos(1,:)
  y : simulink/Sources/Repeating Sequence  rep_seq_t=t  rep_seq_y=BOT3_pos(2,:)
  z : simulink/Sources/Repeating Sequence  rep_seq_t=t  rep_seq_y=BOT3_pos(3,:)
  Conn1 : PMIOPort  Side=Left
  wires:
  y/1 -> Simulink-PS Converter1/1
  x/1 -> Simulink-PS Converter/1
  z/1 -> Subsystem/1(1)
  Subsystem/1(2) -> Simulink-PS Converter2/1
  PS-Simulink Converter1/1 -> Mux/2
  PS-Simulink Converter2/1 -> Mux/3
  PS-Simulink Converter/1 -> Mux/1
  Mux/1 -> Transmitter_BOT3/1
  Pose Estimator Bot4/2(y) -> Mux4/2
  Pose Estimator Bot1/3(z) -> Mux1/3
  Pose Estimator Bot2/2(y) -> Mux2/2
  Pose Estimator Bot1/2(y) -> Mux1/2
  Pose Estimator Bot3/3(z) -> Mux3/3
  Receiver4/4(ed4) -> Pose Estimator Bot4/4(r4t)
  Transmission_Channel/11(Out11) -> Receiver4/11(y4), Receiver3/11(y4), Receiver2/11(y4), Receiver1/11(y4)
  Transmission_Channel/12(Out12) -> Receiver4/12(z4), Receiver3/12(z4), Receiver2/12(z4), Receiver1/12(z4)
  Pose Estimator Bot4/3(z) -> Mux4/3
  Receiver4/2(ed2) -> Pose Estimator Bot2/4(r4t)
  Pose Estimator Bot3/2(y) -> Mux3/2
  Pose Estimator Bot2/1(x) -> Mux2/1
  Pose Estimator Bot2/3(z) -> Mux2/3
  Pose Estimator Bot4/1(x) -> Mux4/1
  Receiver2/4(ed4) -> Pose Estimator Bot4/2(r2t)
  Pose Estimator Bot1/1(x) -> Mux1/1
  Receiver2/2(ed2) -> Pose Estimator Bot2/2(r2t)
  Receiver2/3(ed3) -> Pose Estimator Bot3/2(r2t)
  Receiver3/4(ed4) -> Pose Estimator Bot4/3(r3t)
  Transmission_Channel/3(Out3) -> Receiver4/3(z1), Receiver3/3(z1), Receiver2/3(z1), Receiver1/3(z1)
  Receiver3/3(ed3) -> Pose Estimator Bot3/3(r3t)
  Receiver3/1(ed1) -> Pose Estimator Bot1/3(r3t)
  Pose Estimator Bot3/1(x) -> Mux3/1
  Transmission_Channel/7(Out7) -> Receiver2/7(x3), Receiver4/7(x3), Receiver3/7(x3), Receiver1/7(x3)
  Receiver2/1(ed1) -> Pose Estimator Bot1/2(r2t)
  Receiver1/2(ed2) -> Pose Estimator Bot2/1(r1t)
  Mux4/1 -> LOCAL REGISTER ARRAY 3/4(In4)
  Transmission_Channel/9(Out9) -> Receiver4/9(z3), Receiver3/9(z3), Receiver2/9(z3), Receiver1/9(z3)
  Mux1/1 -> LOCAL REGISTER ARRAY 3/1(In1)
  Transmission_Channel/2(Out2) -> Receiver4/2(y1), Receiver3/2(y1), Receiver2/2(y1), Receiver1/2(y1)
  Transmission_Channel/6(Out6) -> Receiver2/6(z2), Receiver4/6(z2), Receiver3/6(z2), Receiver1/6(z2)
  Receiver1/3(ed3) -> Pose Estimator Bot3/1(r1t)
  Mux2/1 -> LOCAL REGISTER ARRAY 3/2(In2)
  Transmission_Channel/5(Out5) -> Receiver4/5(y2), Receiver3/5(y2), Receiver2/5(y2), Receiver1/5(y2)
  Receiver4/1(ed1) -> Pose Estimator Bot1/4(r4t)
  Transmission_Channel/10(Out10) -> Receiver4/10(x4), Receiver3/10(x4), Receiver2/10(x4), Receiver1/10(x4)
  Transmission_Channel/4(Out4) -> Receiver4/4(x2), Receiver3/4(x2), Receiver2/4(x2), Receiver1/4(x2)
  Receiver1/4(ed4) -> Pose Estimator Bot4/1(r1t)
  Receiver1/1(ed1) -> Pose Estimator Bot1/1(r1t)
  Receiver4/3(ed3) -> Pose Estimator Bot3/4(r4t)
  Mux3/1 -> LOCAL REGISTER ARRAY 3/3(In3)
  Transmission_Channel/8(Out8) -> Receiver4/8(y3), Receiver3/8(y3), Receiver2/8(y3), Receiver1/8(y3)
  Transmission_Channel/1(Out1) -> Receiver1/1(x1), Receiver4/1(x1), Receiver3/1(x1), Receiver2/1(x1)
  Receiver3/2(ed2) -> Pose Estimator Bot2/3(r3t)
  connections:
  BOT3_RIGID/LConn1 -- SixDOF1/RConn1 -- Parallel1/RConn1
  Conn1/RConn1 -- SixDOF1/LConn1 -- Parallel1/LConn1
  SixDOF1/LConn2 -- Simulink-PS Converter/RConn1
  SixDOF1/LConn4 -- Simulink-PS Converter2/RConn1
  SixDOF1/LConn3 -- Simulink-PS Converter1/RConn1
  SixDOF1/RConn4 -- PS-Simulink Converter2/LConn1
  SixDOF1/RConn3 -- PS-Simulink Converter1/LConn1
  SixDOF1/RConn2 -- PS-Simulink Converter/LConn1

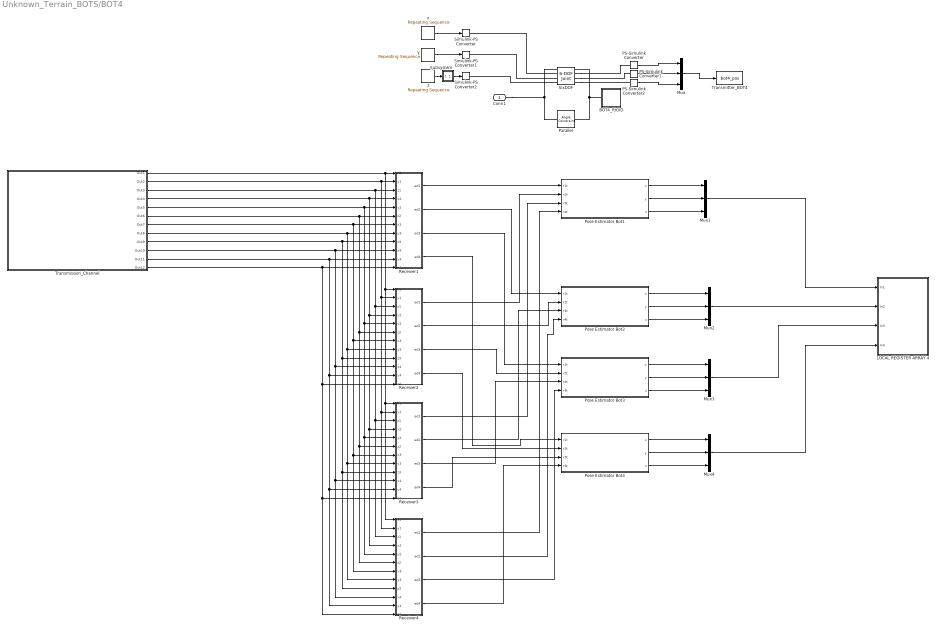
== system Unknown_Terrain_BOTS/BOT4 ==
  BOT4_RIGID : Subsystem
  LOCAL REGISTER ARRAY 4 : Subsystem
  Mux{,1..4} (5 alike) : Mux  Inputs=3
  PS-Simulink Converter : nesl_utility/PS-Simulink Converter  PhysicalDomain=network_engine_domain  SubClassName=ps_output  LeftPortType=input  RightPortType=output  PseudoPeriodic=off  Frequencies=[]  Unit=m  AffineConversion=off
  PS-Simulink Converter1 : nesl_utility/PS-Simulink Converter  PhysicalDomain=network_engine_domain  SubClassName=ps_output  LeftPortType=input  RightPortType=output  PseudoPeriodic=off  Frequencies=[]  Unit=m  AffineConversion=off
  PS-Simulink Converter2 : nesl_utility/PS-Simulink Converter  PhysicalDomain=network_engine_domain  SubClassName=ps_output  LeftPortType=input  RightPortType=output  PseudoPeriodic=off  Frequencies=[]  Unit=m  AffineConversion=off
  Parallel : sm_lib/Constraints/Angle Constraint  ConstraintType=Parallel  Angle=45  AngleUnits=deg  SenseSignedTorqueMagnitude=off  SenseTorque=off  SenseForce=off  WrenchDir=FollowerOnBase  WrenchFrame=BaseFrame
      settings: SourceProductName=Simscape Multibody  SourceProductBaseCode=MS
  Pose Estimator Bot1 : MATLAB Function  TreatAsAtomicUnit=on
  Pose Estimator Bot2 : MATLAB Function  TreatAsAtomicUnit=on
  Pose Estimator Bot3 : MATLAB Function  TreatAsAtomicUnit=on
  Pose Estimator Bot4 : MATLAB Function  TreatAsAtomicUnit=on
  Receiver1 : MATLAB Function  TreatAsAtomicUnit=on
  Receiver2 : MATLAB Function  TreatAsAtomicUnit=on
  Receiver3 : MATLAB Function  TreatAsAtomicUnit=on
  Receiver4 : MATLAB Function  TreatAsAtomicUnit=on
  Simulink-PS Converter : nesl_utility/Simulink-PS Converter  PhysicalDomain=network_engine_domain  SubClassName=ps_input  LeftPortType=input  RightPortType=output  PseudoPeriodic=off  Frequencies=[]  NoiseDistribution=none  NoiseParameters=[]  Unit=m  AffineConversion=off  FilteringAndDerivatives=filter  SimscapeFilterOrder=2  InputFilterTimeConstant=0.001  UdotUserProvided=0
  Simulink-PS Converter1 : nesl_utility/Simulink-PS Converter  PhysicalDomain=network_engine_domain  SubClassName=ps_input  LeftPortType=input  RightPortType=output  PseudoPeriodic=off  Frequencies=[]  NoiseDistribution=none  NoiseParameters=[]  Unit=m  AffineConversion=off  FilteringAndDerivatives=filter  SimscapeFilterOrder=2  InputFilterTimeConstant=0.001  UdotUserProvided=0
  Simulink-PS Converter2 : nesl_utility/Simulink-PS Converter  PhysicalDomain=network_engine_domain  SubClassName=ps_input  LeftPortType=input  RightPortType=output  PseudoPeriodic=off  Frequencies=[]  NoiseDistribution=none  NoiseParameters=[]  Unit=m  AffineConversion=off  FilteringAndDerivatives=filter  SimscapeFilterOrder=2  InputFilterTimeConstant=0.001  UdotUserProvided=0
  SixDOF : sm_lib/Joints/6-DOF Joint  SenseConstraintForce=off  SenseConstraintForceX=off  SenseConstraintForceY=off  SenseConstraintForceZ=off  SenseConstraintTorque=off  SenseConstraintTorqueX=off  SenseConstraintTorqueY=off  SenseConstraintTorqueZ=off  SenseTotalForce=off  SenseTotalForceX=off  SenseTotalForceY=off  SenseTotalForceZ=off  SenseTotalTorque=off  SenseTotalTorqueX=off  SenseTotalTorqueY=off  SenseTotalTorqueZ=off  CompositeWrenchDir=FollowerOnBase  CompositeWrenchFrame=BaseFrame  PxEquilibriumPosition=0  PxEquilibriumPositionUnits=m  PxSpringStiffness=0  PxSpringStiffnessUnits=N/m  PxDampingCoefficient=0  PxDampingCoefficientUnits=N/(m/s)  PxTorqueActuationMode=ComputedTorque  PxMotionActuationMode=InputMotion  PxSensePosition=on  PxSenseVelocity=off  PxSenseAcceleration=off  PxSenseTorqueForce=off  PxPositionTargetSpecify=on  PxPositionTargetPriority=Low  PxPositionTargetValue=smiData.SixDofJoint(1).Px.Pos  PxPositionTargetValueUnits=in  PxVelocityTargetSpecify=off  PxVelocityTargetPriority=High  PxVelocityTargetValue=0  PxVelocityTargetValueUnits=m/s  PyEquilibriumPosition=0  PyEquilibriumPositionUnits=m  PySpringStiffness=0  PySpringStiffnessUnits=N/m  PyDampingCoefficient=0  PyDampingCoefficientUnits=N/(m/s)  PyTorqueActuationMode=ComputedTorque  PyMotionActuationMode=InputMotion  PySensePosition=on  PySenseVelocity=off  PySenseAcceleration=off  PySenseTorqueForce=off  PyPositionTargetSpecify=on  PyPositionTargetPriority=Low  PyPositionTargetValue=smiData.SixDofJoint(1).Py.Pos  PyPositionTargetValueUnits=in  PyVelocityTargetSpecify=off  PyVelocityTargetPriority=High  PyVelocityTargetValue=0  PyVelocityTargetValueUnits=m/s  PzEquilibriumPosition=0  PzEquilibriumPositionUnits=m  PzSpringStiffness=0  PzSpringStiffnessUnits=N/m  PzDampingCoefficient=0  PzDampingCoefficientUnits=N/(m/s)  PzTorqueActuationMode=ComputedTorque  PzMotionActuationMode=InputMotion  PzSensePosition=on  PzSenseVelocity=off  PzSenseAcceleration=off  PzSenseTorqueForce=off  PzPositionTargetSpecify=on  PzPositionTargetPriority=Low  PzPositionTargetValue=smiData.SixDofJoint(1).Pz.Pos  PzPositionTargetValueUnits=in  PzVelocityTargetSpecify=off  PzVelocityTargetPriority=High  PzVelocityTargetValue=0  PzVelocityTargetValueUnits=m/s  SphDefPosRotationMethod=None  SphDefPosRotationAngleUnits=deg  SphDefPosRotationStandardAxis=+Z  SphDefPosRotationAngle=0.0  SphDefPosRotationArbitraryAxis=[0 0 1]  SphDefPosFollAlignAxisA=+X  SphDefPosBaseAlignAxisA=+Y  SphDefPosFollAlignAxisB=+Y  SphDefPosBaseAlignAxisB=+Z  SphDefPosRotationSequenceAxes=FollowerAxes  SphDefPosRotationSequence=XYX  SphDefPosRotationSequenceAngles=[0 0 0]  SphDefPosRotationSequenceAnglesUnits=deg  SphDefPosRotationMatrix=[1 0 0; 0 1 0; 0 0 1]  SphEqPosRotationMethod=None  SphEqPosRotationAngleUnits=deg  SphEqPosRotationStandardAxis=+Z  SphEqPosRotationAngle=0.0  SphEqPosRotationArbitraryAxis=[0 0 1]  SphEqPosFollAlignAxisA=+X  SphEqPosBaseAlignAxisA=+Y  SphEqPosFollAlignAxisB=+Y  SphEqPosBaseAlignAxisB=+Z  SphEqPosRotationSequenceAxes=FollowerAxes  SphEqPosRotationSequence=XYX  SphEqPosRotationSequenceAngles=[0 0 0]  SphEqPosRotationSequenceAnglesUnits=deg  SphEqPosRotationMatrix=[1 0 0; 0 1 0; 0 0 1]  SphSpringStiffness=0  SphSpringStiffnessUnits=N*m/rad  SphDampingCoefficient=0  SphDampingCoefficientUnits=N*m/(rad/s)  SphActuateTorqueX=off  SphActuateTorqueY=off  SphActuateTorqueZ=off  SphActuateTorque=off  SphTorqueActuationMode=NoTorque  SphMotionActuationMode=ComputedMotion  SphActuationFrame=BaseFrame  SphSensePosition=off  SphSenseVelocityX=off  SphSenseVelocityY=off  SphSenseVelocityZ=off  SphSenseVelocity=off  SphSenseAccelerationX=off  SphSenseAccelerationY=off  SphSenseAccelerationZ=off  SphSenseAcceleration=off  SphSenseTorqueX=off  SphSenseTorqueY=off  SphSenseTorqueZ=off  SphSenseTorqueForce=off  SphSensingFrame=FollowerFrame  SphPositionTargetRotationMethod=ArbitraryAxis  SphPositionTargetRotationAngleUnits=deg  SphPositionTargetRotationStandardAxis=+Z  SphPositionTargetRotationAngle=smiData.SixDofJoint(1).S.Pos.Angle  SphPositionTargetRotationArbitraryAxis=smiData.SixDofJoint(1).S.Pos.Axis  SphPositionTargetFollAlignAxisA=+X  SphPositionTargetBaseAlignAxisA=+Y  SphPositionTargetFollAlignAxisB=+Y  SphPositionTargetBaseAlignAxisB=+Z  SphPositionTargetRotationSequenceAxes=FollowerAxes  SphPositionTargetRotationSequence=XYX  SphPositionTargetRotationSequenceAngles=[0 0 0]  SphPositionTargetRotationSequenceAnglesUnits=deg  SphPositionTargetRotationMatrix=[1 0 0; 0 1 0; 0 0 1]  SphPositionTargetSpecify=on  SphPositionTargetPriority=Low  SphVelocityTargetValue=[0 0 0]  SphVelocityTargetValueUnits=deg/s  SphVelocityTargetSpecify=off  SphVelocityTargetPriority=High  SphVelocityTargetInFollowerFrame=on
  Subsystem : Subsystem
  Transmission_Channel : Subsystem
  Transmitter_BOT4 : ToWorkspace  VariableName=bot4_pos  SampleTime=-1
  x : simulink/Sources/Repeating Sequence  rep_seq_t=t  rep_seq_y=BOT4_pos(1,:)
  y : simulink/Sources/Repeating Sequence  rep_seq_t=t  rep_seq_y=BOT4_pos(2,:)
  z : simulink/Sources/Repeating Sequence  rep_seq_t=t  rep_seq_y=BOT4_pos(3,:)
  Conn1 : PMIOPort  Side=Left
  wires:
  z/1 -> Subsystem/1(1)
  y/1 -> Simulink-PS Converter1/1
  x/1 -> Simulink-PS Converter/1
  Subsystem/1(2) -> Simulink-PS Converter2/1
  PS-Simulink Converter1/1 -> Mux/2
  PS-Simulink Converter2/1 -> Mux/3
  PS-Simulink Converter/1 -> Mux/1
  Mux/1 -> Transmitter_BOT4/1
  Pose Estimator Bot4/2(y) -> Mux4/2
  Pose Estimator Bot1/3(z) -> Mux1/3
  Pose Estimator Bot2/2(y) -> Mux2/2
  Pose Estimator Bot1/2(y) -> Mux1/2
  Pose Estimator Bot3/3(z) -> Mux3/3
  Receiver4/4(ed4) -> Pose Estimator Bot4/4(r4t)
  Transmission_Channel/11(Out11) -> Receiver4/11(y4), Receiver3/11(y4), Receiver2/11(y4), Receiver1/11(y4)
  Transmission_Channel/12(Out12) -> Receiver4/12(z4), Receiver3/12(z4), Receiver2/12(z4), Receiver1/12(z4)
  Pose Estimator Bot4/3(z) -> Mux4/3
  Receiver4/2(ed2) -> Pose Estimator Bot2/4(r4t)
  Pose Estimator Bot3/2(y) -> Mux3/2
  Pose Estimator Bot2/1(x) -> Mux2/1
  Pose Estimator Bot2/3(z) -> Mux2/3
  Pose Estimator Bot4/1(x) -> Mux4/1
  Receiver2/4(ed4) -> Pose Estimator Bot4/2(r2t)
  Pose Estimator Bot1/1(x) -> Mux1/1
  Receiver2/2(ed2) -> Pose Estimator Bot2/2(r2t)
  Receiver2/3(ed3) -> Pose Estimator Bot3/2(r2t)
  Receiver3/4(ed4) -> Pose Estimator Bot4/3(r3t)
  Transmission_Channel/3(Out3) -> Receiver4/3(z1), Receiver3/3(z1), Receiver2/3(z1), Receiver1/3(z1)
  Receiver3/3(ed3) -> Pose Estimator Bot3/3(r3t)
  Receiver3/1(ed1) -> Pose Estimator Bot1/3(r3t)
  Pose Estimator Bot3/1(x) -> Mux3/1
  Transmission_Channel/7(Out7) -> Receiver2/7(x3), Receiver4/7(x3), Receiver3/7(x3), Receiver1/7(x3)
  Receiver2/1(ed1) -> Pose Estimator Bot1/2(r2t)
  Receiver1/2(ed2) -> Pose Estimator Bot2/1(r1t)
  Mux4/1 -> LOCAL REGISTER ARRAY 4/4(In4)
  Transmission_Channel/9(Out9) -> Receiver4/9(z3), Receiver3/9(z3), Receiver2/9(z3), Receiver1/9(z3)
  Mux1/1 -> LOCAL REGISTER ARRAY 4/1(In1)
  Transmission_Channel/2(Out2) -> Receiver4/2(y1), Receiver3/2(y1), Receiver2/2(y1), Receiver1/2(y1)
  Transmission_Channel/6(Out6) -> Receiver2/6(z2), Receiver4/6(z2), Receiver3/6(z2), Receiver1/6(z2)
  Receiver1/3(ed3) -> Pose Estimator Bot3/1(r1t)
  Mux2/1 -> LOCAL REGISTER ARRAY 4/2(In2)
  Transmission_Channel/5(Out5) -> Receiver4/5(y2), Receiver3/5(y2), Receiver2/5(y2), Receiver1/5(y2)
  Receiver4/1(ed1) -> Pose Estimator Bot1/4(r4t)
  Transmission_Channel/10(Out10) -> Receiver4/10(x4), Receiver3/10(x4), Receiver2/10(x4), Receiver1/10(x4)
  Transmission_Channel/4(Out4) -> Receiver4/4(x2), Receiver3/4(x2), Receiver2/4(x2), Receiver1/4(x2)
  Receiver1/4(ed4) -> Pose Estimator Bot4/1(r1t)
  Receiver1/1(ed1) -> Pose Estimator Bot1/1(r1t)
  Receiver4/3(ed3) -> Pose Estimator Bot3/4(r4t)
  Mux3/1 -> LOCAL REGISTER ARRAY 4/3(In3)
  Transmission_Channel/8(Out8) -> Receiver4/8(y3), Receiver3/8(y3), Receiver2/8(y3), Receiver1/8(y3)
  Transmission_Channel/1(Out1) -> Receiver1/1(x1), Receiver4/1(x1), Receiver3/1(x1), Receiver2/1(x1)
  Receiver3/2(ed2) -> Pose Estimator Bot2/3(r3t)
  connections:
  Conn1/RConn1 -- SixDOF/LConn1 -- Parallel/LConn1
  Parallel/RConn1 -- BOT4_RIGID/LConn1 -- SixDOF/RConn1
  SixDOF/LConn3 -- Simulink-PS Converter1/RConn1
  SixDOF/LConn2 -- Simulink-PS Converter/RConn1
  SixDOF/LConn4 -- Simulink-PS Converter2/RConn1
  SixDOF/RConn4 -- PS-Simulink Converter2/LConn1
  SixDOF/RConn3 -- PS-Simulink Converter1/LConn1
  SixDOF/RConn2 -- PS-Simulink Converter/LConn1

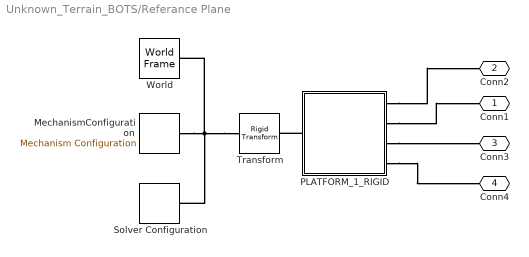
== system Unknown_Terrain_BOTS/Referance Plane ==
  MechanismConfiguration : sm_lib/Utilities/Mechanism Configuration  UniformGravity=Constant  GravityVector=[0 -9.80665 0]  GravityUnits=m/s^2  LinearizationDelta=0.001
  PLATFORM_1_RIGID : Subsystem
  Solver Configuration : nesl_utility/Solver Configuration  PhysicalDomain=network_engine_domain  SubClassName=solver  LeftPortType=input  RightPortType=generic  Tones=[]  Harmonics=[]  SimulateNoise=off  Profile=off  UseLocalSampling=off  EnableSwitchedLinearOptims=on  FrequencyDomain=off  UseCCode=off  RelTol=0.001  AbsTol=1e-06  MinStep=1e-09  ToWorkspace=off  RevertToSquareIcSolve=off  NumHomotopyIterations=100  PhasorMode=off  PhasorModeNumHarmonics=1  DoDC=off  ResidualTolerance=1e-09  UseLocalSolver=off  LocalSolverChoice=NE_BACKWARD_EULER_ADVANCER  LocalSolverSampleTime=0.001  DoFixedCost=off  MaxNonlinIter=3  MaxModeIter=2  LinearAlgebra=auto  EquationFormulation=NE_TIME_EF  DelaysMemoryBudget=1024  AutomaticFiltering=on  FilteringTimeConstant=0.001  PartitionStorageMethod=AS_NEEDED  PartitionMemoryBudget=1024
  Transform : sm_lib/Frames and Transforms/Rigid Transform  TranslationMethod=Cartesian  TranslationStandardOffset=0  TranslationLengthUnit=m  TranslationStandardAxis=+Z  TranslationCartesianOffset=smiData.RigidTransform(9).translation  TranslationROffset=0  TranslationROffsetUnits=m  TranslationZOffset=0  TranslationZOffsetUnits=m  TranslationThetaOffset=0  TranslationThetaOffsetUnits=deg  RotationMethod=ArbitraryAxis  RotationAngleUnits=rad  RotationStandardAxis=+Z  RotationAngle=smiData.RigidTransform(9).angle  RotationArbitraryAxis=smiData.RigidTransform(9).axis  FollAlignAxisA=+X  BaseAlignAxisA=+Y  FollAlignAxisB=+Y  BaseAlignAxisB=+Z  RotationSequenceAxes=FollowerAxes  RotationSequence=XYX  RotationSequenceAngles=[0 0 0]  RotationSequenceAnglesUnits=deg  RotationMatrix=[1 0 0; 0 1 0; 0 0 1]
  World : sm_lib/Frames and Transforms/World Frame
  Conn1 : PMIOPort  Side=Right
  Conn2 : PMIOPort  Port=2  Side=Right
  Conn3 : PMIOPort  Port=3  Side=Right
  Conn4 : PMIOPort  Port=4  Side=Right
  connections:
  PLATFORM_1_RIGID/RConn3 -- Conn3/RConn1
  Transform/LConn1 -- MechanismConfiguration/RConn1 -- Solver Configuration/RConn1 -- World/RConn1
  PLATFORM_1_RIGID/LConn1 -- Transform/RConn1
  PLATFORM_1_RIGID/RConn1 -- Conn2/RConn1
  PLATFORM_1_RIGID/RConn4 -- Conn4/RConn1
  PLATFORM_1_RIGID/RConn2 -- Conn1/RConn1
